simulink model "linearModel"  (R2017a)
settings: Solver=VariableStepAuto  StartTime=0.0  StopTime=60  RelTol=1e-3
undefined symbols (not defined in the file): LIN_AC_S_A, LIN_AC_S_B, LIN_AC_S_C, LIN_AC_S_D, ss6
settings Model: Creator=abemart  LastModifiedBy=hbolandhemmat

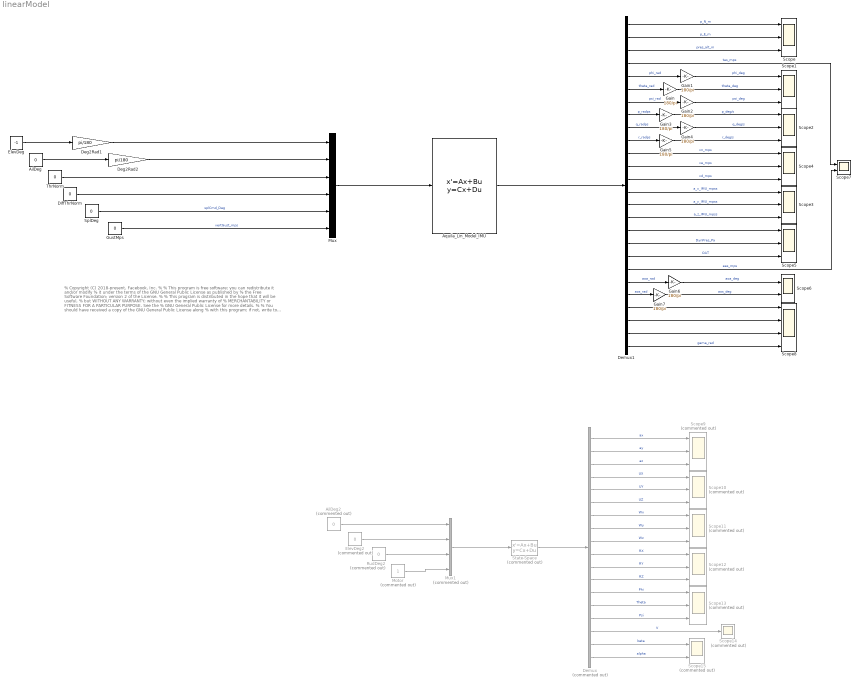
== system linearModel ==
  note: % Copyright (C) 2018-present, Facebook, Inc.
      | %
      | % This program is free software; you can redistribute it and/or modify
      | % it under the terms of the GNU General Public License as published by
      | % the Free Software Foundation; version 2 of the License.
      | %
      | % This program is distributed in the hope that it will be useful,
      | % but WITHOUT ANY WARRANTY; without even the implied warranty of
      | % MERCHANTABILITY or FITNESS FOR A PARTICULAR PURPOSE. See the
      | % GNU General Public License for more details.
      | %
      | % You should have received a copy of the GNU General Public License along
      | % with this program; if not, write to the Free Software Foundation, Inc.,
      | % 51 Franklin Street, Fifth Floor, Boston, MA 02110-1301 USA.
  AilDeg : Constant  Value=0
  AilDeg2 : Constant  Commented=on  Value=0
  Aquila_Lin_Model_IMU : StateSpace  A=LIN_AC_S_A  B=LIN_AC_S_B  C=LIN_AC_S_C  D=LIN_AC_S_D  X0=0
  Deg2Rad1 : Gain  Gain=pi/180
  Deg2Rad2 : Gain  Gain=pi/180
  Demux : Demux  Commented=on  Outputs=18
  Demux1 : Demux  Outputs=26
  "DiffThrNorm " : Constant  Value=0
  "ElevDeg " : Constant  Value=-1
  ElevDeg2 : Constant  Commented=on  Value=0
  Gain{,1..7} (8 alike) : Gain  Gain=180/pi
  GustMps : Constant  Value=0
  Motor : Constant  Commented=on
  Mux : Mux  Inputs=6
  Mux1 : Mux  Commented=on
  RudDeg2 : Constant  Commented=on  Value=0
  Scope{,1..5} (6 alike) : Scope  NumInputPorts=3
  Scope{9..13} (5 alike) : Scope  Commented=on  NumInputPorts=3
  Scope14 : Scope  Commented=on
  Scope15 : Scope  Commented=on  NumInputPorts=2
  Scope6 : Scope  NumInputPorts=2
  Scope7 : Scope  NumInputPorts=2
  Scope8 : Scope  NumInputPorts=4
  SplDeg : Constant  Value=0
  State-Space : StateSpace  Commented=on  A=ss6.A  B=ss6.B  C=ss6.C  D=ss6.D  X0=0
  ThrNorm : Constant  Value=0
  wires:
  Mux/1 -> Aquila_Lin_Model_IMU/1
  Demux1/13 -> Scope4/3  "vd_mps"
  Demux1/12 -> Scope4/2  "ve_mps"
  Demux1/11 -> Scope4/1  "vn_mps"
  Demux1/25 -> Scope8/3
  Demux1/10 -> Gain5/1  "r_radps"
  Demux1/26 -> Scope8/4  "gama_rad"
  Demux1/24 -> Scope8/2
  Demux1/23 -> Scope8/1
  Demux1/22 -> Gain7/1  "aos_rad"
  Demux1/21 -> Gain6/1  "aoa_rad"
  Demux1/20 -> Scope7/2  "eas_mps"
  Demux1/4 -> Scope7/1  "tas_mps"
  Aquila_Lin_Model_IMU/1 -> Demux1/1
  Demux1/9 -> Gain4/1  "q_radps"
  Demux1/6 -> Gain/1  "theta_rad"
  Demux1/7 -> Gain2/1  "psi_rad"
  Demux1/16 -> Scope3/3  "a_z_IMU_mpss"
  Demux1/14 -> Scope3/1  "a_x_IMU_mpss"
  Demux1/5 -> Gain1/1  "phi_rad"
  Demux1/19 -> Scope5/3  "OAT"
  Demux1/1 -> Scope/1  "p_N_m"
  Demux1/17 -> Scope5/1
  Demux1/18 -> Scope5/2  "DynPres_Pa"
  Demux1/2 -> Scope/2  "p_E_m"
  Demux1/3 -> Scope/3  "pres_alt_m"
  Demux1/15 -> Scope3/2  "a_y_IMU_mpss"
  Demux1/8 -> Gain3/1  "p_radps"
  Mux1/1 -> State-Space/1
  State-Space/1 -> Demux/1
  Demux/1 -> Scope9/1  "ax"
  Demux/2 -> Scope9/2  "ay"
  Demux/3 -> Scope9/3  "az"
  Demux/4 -> Scope10/1  "UX"
  Demux/5 -> Scope10/2  "UY"
  Demux/6 -> Scope10/3  "UZ"
  Demux/7 -> Scope11/1  "Wx"
  Demux/8 -> Scope11/2  "Wy"
  Demux/9 -> Scope11/3  "Wz"
  Demux/10 -> Scope12/1  "RX"
  Demux/11 -> Scope12/2  "RY"
  Demux/12 -> Scope12/3  "RZ"
  Demux/13 -> Scope13/1  "Phi"
  Demux/14 -> Scope13/2  "Theta"
  Demux/15 -> Scope13/3  "Psi"
  Demux/16 -> Scope14/1  "V"
  Demux/17 -> Scope15/1  "beta"
  Demux/18 -> Scope15/2  "alpha"
  SplDeg/1 -> Mux/5  "splCmd_Deg"
  "DiffThrNorm "/1 -> Mux/4
  Deg2Rad1/1 -> Mux/1
  GustMps/1 -> Mux/6  "vertGust_mps"
  Deg2Rad2/1 -> Mux/2
  "ElevDeg "/1 -> Deg2Rad1/1
  AilDeg/1 -> Deg2Rad2/1
  AilDeg2/1 -> Mux1/1
  ElevDeg2/1 -> Mux1/2
  RudDeg2/1 -> Mux1/3
  Motor/1 -> Mux1/4
  ThrNorm/1 -> Mux/3
  Gain/1 -> Scope1/2  "theta_deg"
  Gain1/1 -> Scope1/1  "phi_deg"
  Gain2/1 -> Scope1/3  "psi_deg"
  Gain3/1 -> Scope2/1  "p_deg/s"
  Gain4/1 -> Scope2/2  "q_deg/s"
  Gain5/1 -> Scope2/3  "r_deg/s"
  Gain6/1 -> Scope6/1  "aoa_deg"
  Gain7/1 -> Scope6/2  "aos_deg"
